simulink model "test3"  (R2015a)
settings: Solver=ode45  StartTime=0.0  StopTime=100000000  RelTol=1e-3
libraries: simulink_extras x1
settings Model: Creator=kkhoo  LastModifiedBy=kkhoo

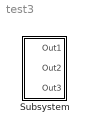
== system test3 ==
  Subsystem : Subsystem

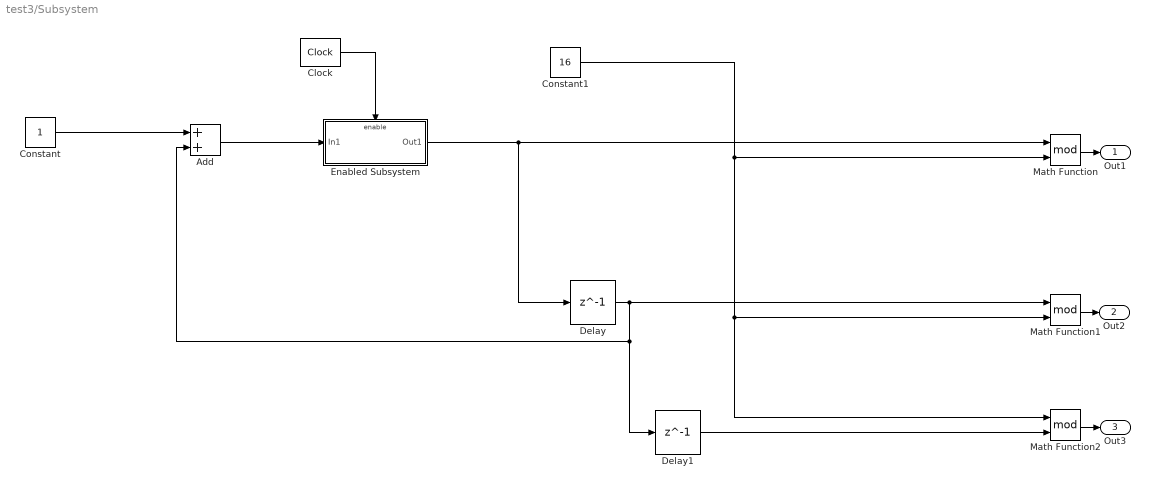
== system test3/Subsystem ==
  Add : Sum
  Clock : simulink_extras/Flip Flops/Clock  period=1000000
  Constant : Constant
  Constant1 : Constant  Value=16
  Delay : Delay  DelayLength=1  InitialCondition=0
  Delay1 : Delay  DelayLength=1  InitialCondition=0
  Enabled Subsystem : Subsystem  TreatAsAtomicUnit=on
  Math Function : Math  Operator=mod  SaturateOnIntegerOverflow=on
  Math Function1 : Math  Operator=mod  SaturateOnIntegerOverflow=on
  Math Function2 : Math  Operator=mod  SaturateOnIntegerOverflow=on
  Out1 : Outport
  Out2 : Outport  Port=2
  Out3 : Outport  Port=3
  wires:
  Enabled Subsystem/1(Out1) -> Math Function/1, Delay/1
  Clock/1 -> Enabled Subsystem/Enable
  Constant/1 -> Add/1
  Math Function/1 -> Out1/1
  Math Function2/1 -> Out3/1
  Delay1/1 -> Math Function2/2
  Math Function1/1 -> Out2/1
  Add/1 -> Enabled Subsystem/1(In1)
  Constant1/1 -> Math Function/2, Math Function2/1, Math Function1/2
  Delay/1 -> Delay1/1, Add/2, Math Function1/1

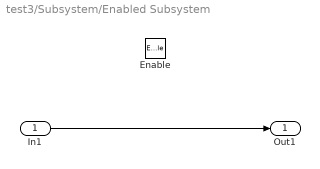
== system test3/Subsystem/Enabled Subsystem ==
  In1 : Inport
  Enable : EnablePort
  Out1 : Outport
  wires:
  In1/1 -> Out1/1
